simulink model "MotionController_mod"  (Simulink 7.6)
settings: Solver=FixedStepDiscrete  SolverMode=SingleTasking  StartTime=0.0  StopTime=inf  FixedStep=0.02  RelTol=1e-3  SampleTimeConstraint=Specified
undefined symbols (not defined in the file): Compass_Yaw_Kd, Compass_Yaw_Ki, Compass_Yaw_Kp, Depth_Kd, Depth_Ki, Depth_Kp, DiscIntNeverNeededParam, IMU_YawRate_Kd, IMU_YawRate_Ki, IMU_YawRate_Kp, IMU_YVel_Kd, IMU_YVel_Ki, IMU_YVel_Kp, Target_Down_X_Kd, Target_Down_X_Ki, Target_Down_X_Kp, Target_Down_Y_Kd, Target_Down_Y_Ki, Target_Down_Y_Kp, Target_Down_Yaw_Kd, Target_Down_Yaw_Ki, Target_Down_Yaw_Kp, Target_Forward_Y_Kd, Target_Forward_Y_Ki, Target_Forward_Y_Kp, Target_Forward_Yaw_Kd, Target_Forward_Yaw_Ki, Target_Forward_Yaw_Kp, Target_Forward_Z_Kd, Target_Forward_Z_Ki, Target_Forward_Z_Kp, Thruster_Friction_Zero, Thruster_LeftAngled_Gain, Thruster_LeftFwd_Gain, Thruster_RightAngled_Gain, Thruster_RightFwd_Gain, ZVelocity_Neg_Max
libraries: simulink x13, libAUVT x6, neural x1
settings Model: Creator=auvt  LastModifiedBy=auvt  ParamWorkspaceSource=ReferencedWorkspace  TunableVars=Compass_Yaw_Kd,Compass_Yaw_Ki,Compass_Yaw_Kp,Depth_Kd,Depth_Ki,Depth_Kp,Heading_Kd,Heading_Ki,Heading_Kp,IMU_YVel_Kd,IMU_YVel_Ki,IMU_YVel_Kp,IMU_YawRate_Kd,IMU_YawRate_Ki,IMU_YawRate_Kp,Target_Down_X_Kd,Target_Down_X_Ki,Target_Down_X_Kp,Target_Down_Y_Kd,Target_Down_Y_Ki,Target_Down_Y_Kp,Target_Down_Yaw_Kd,Target_Down_Yaw_Ki,Target_Down_Yaw_Kp,Target_Forward_Y_Kd,Target_Forward_Y_Ki,Target_Forward_Y_Kp,Target_Forward_Yaw_Kd,Target_Forward_Yaw_Ki,Target_Forward_Yaw_Kp,Target_Forward_Z_Kd,Target_Forward_Z_Ki,Target_Forward_Z_Kp,Thruster_Friction_Zero,Thruster_LeftAngled_Gain,Thruster_LeftFwd_Gain,Thruster_RightAngled_Gain,Thruster_RightFwd_Gain,ZVelocity_Neg_Max  TunableVarsStorageClass=Auto,Auto,Auto,Auto,Auto,Auto,Auto,Auto,Auto,Auto,Auto,Auto,Auto,Auto,Auto,Auto,Auto,Auto,Auto,Auto,Auto,Auto,Auto,Auto,Auto,Auto,Auto,Auto,Auto,Auto,Auto,Auto,Auto,Auto,Auto,Auto,Auto,Auto,Auto  TunableVarsTypeQualifier=,,,,,,,,,,,,,,,,,,,,,,,,,,,,,,,,,,,,,,
settings MATStruct: SampleTime=0.02  Offset=0  Priority=[1.0]
settings OptimizationCC: InlineParams=on  OptimizeModelRefInitCode=on  LifeSpan=1
settings RTWCC: SystemTargetFile=ert.tlc  GenCodeOnly=on  TemplateMakefile=ert_default_tmf  PostCodeGenCommand=packNGo(buildInfo);  Description=Real-Time Workshop Embedded Coder  GenerateReport=on  ProcessScript=ert_make_rtw_hook  IncludeHyperlinkInReport=on  LaunchReport=on  TargetLang=C++
settings CodeAppCC: IgnoreCustomStorageClasses=off
settings ERTTargetCC: MultiwordLength=2048  GenerateSampleERTMain=on  IncludeMdlTerminateFcn=off  InlinedParameterPlacement=NonHierarchical  ERTCustomFileTemplate=example_file_process.tlc  ConvertIfToSwitch=off

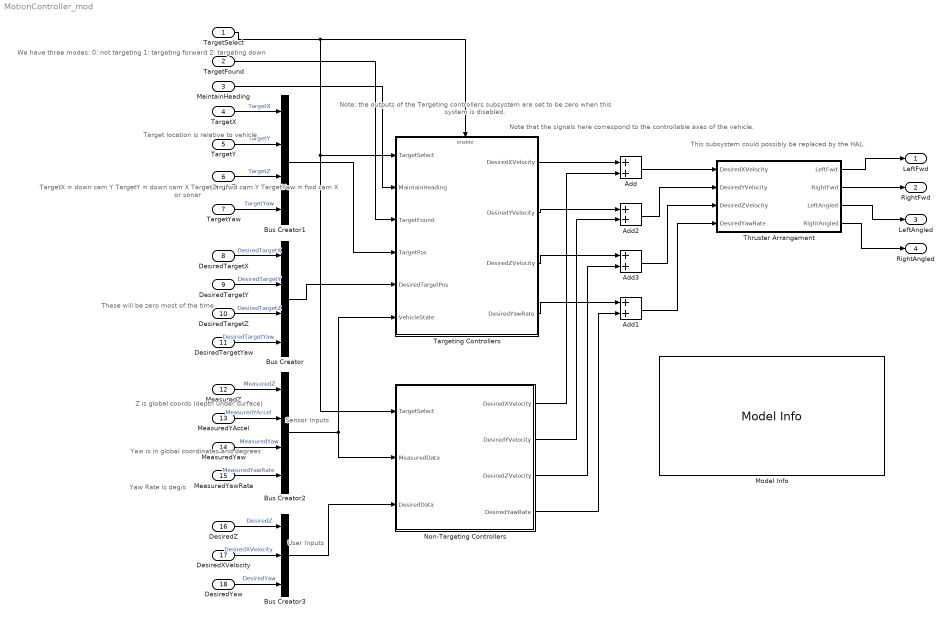
== system MotionController_mod ==
  note: We have three modes:
      |  0: not targeting
      | 1: targeting forward
      | 2: targeting down
  note: Target location
      | is relative to
      | vehicle
  note: Yaw is in global
      | coordinates
      | and degrees
  note: Yaw Rate is deg/s
  note: These will be zero
      | most of the time
  note: Z is global coords
      | (depth under surface)
  note: TargetX = down cam Y
      | TargetY = down cam X
      | TargetZ = fwd cam Y
      | TargetYaw = fwd cam X
      | or sonar
  note: This subsystem could possibly
      |  be replaced by the HAL.
  note: Note that the signals here correspond
      | to the controllable axes of the vehicle.
  note: Sensor
      | Inputs
  note: User
      | Inputs
  note: Note: the outputs of the Targeting controllers
      | subsystem are set to be zero when this
      | system is disabled.
  TargetSelect : Inport  SampleTime=0.02
  TargetFound : Inport  Port=2  SampleTime=0.02
  MaintainHeading : Inport  Port=3
  TargetX : Inport  Port=4
  TargetY : Inport  Port=5
  TargetZ : Inport  Port=6
  TargetYaw : Inport  Port=7
  DesiredTargetX : Inport  Port=8
  DesiredTargetY : Inport  Port=9
  DesiredTargetZ : Inport  Port=10
  DesiredTargetYaw : Inport  Port=11
  MeasuredZ : Inport  Port=12  SampleTime=0.02
  MeasuredYAccel : Inport  Port=13  SampleTime=0.02
  MeasuredYaw : Inport  Port=14  SampleTime=0.02
  MeasuredYawRate : Inport  Port=15
  DesiredZ : Inport  Port=16
  DesiredXVelocity : Inport  Port=17
  DesiredYaw : Inport  Port=18
  Add{,1..3} (4 alike) : Sum
  Bus Creator : BusCreator
  Bus Creator1 : BusCreator
  Bus Creator2 : BusCreator
  Bus Creator3 : BusCreator  Inputs=3
  Model Info : simulink/Model-Wide Utilities/Model Info  SystemSampleTime=-1  InitialBlockCM=None  BlockCM=None  Frame=on  DisplayStringWithTags=|  HorizontalTextAlignment=Left  LeftAlignmentValue=0.02  SourceBlockDiagram=MotionController_mod  TagMaxNumber=20
      | This Model directly controls the
      |  thrusters by using several controllers. 
      |  The controllers are based on current
      |  state information (heading, depth, etc.)
      |  as well as desired state info.
      | 
      | %<LastModifiedBy>
      | %<LastModificationDate>
  Non-Targeting Controllers : Subsystem
  Targeting Controllers : Subsystem  TreatAsAtomicUnit=on
  Thruster Arrangement : Subsystem
  LeftFwd : Outport
  RightFwd : Outport  Port=2
  LeftAngled : Outport  Port=3
  RightAngled : Outport  Port=4
  wires:
  Thruster Arrangement/1(LeftFwd) -> LeftFwd/1
  Thruster Arrangement/2(RightFwd) -> RightFwd/1
  Thruster Arrangement/3(LeftAngled) -> LeftAngled/1
  Thruster Arrangement/4(RightAngled) -> RightAngled/1
  TargetSelect/1 -> Targeting Controllers/Enable, Non-Targeting Controllers/1(TargetSelect), Targeting Controllers/1(TargetSelect)
  TargetFound/1 -> Targeting Controllers/3(TargetFound)
  Add/1 -> Thruster Arrangement/1(DesiredXVelocity)
  Add1/1 -> Thruster Arrangement/4(DesiredYawRate)
  Add2/1 -> Thruster Arrangement/2(DesiredYVelocity)
  Add3/1 -> Thruster Arrangement/3(DesiredZVelocity)
  Targeting Controllers/1(DesiredXVelocity) -> Add/1
  Targeting Controllers/4(DesiredYawRate) -> Add1/1
  Targeting Controllers/2(DesiredYVelocity) -> Add2/1
  Targeting Controllers/3(DesiredZVelocity) -> Add3/1
  Non-Targeting Controllers/2(DesiredYVelocity) -> Add2/2
  Non-Targeting Controllers/4(DesiredYawRate) -> Add1/2
  Non-Targeting Controllers/3(DesiredZVelocity) -> Add3/2
  DesiredTargetX/1 -> Bus Creator/1  "DesiredTargetX"
  DesiredTargetY/1 -> Bus Creator/2  "DesiredTargetY"
  DesiredTargetZ/1 -> Bus Creator/3  "DesiredTargetZ"
  DesiredTargetYaw/1 -> Bus Creator/4  "DesiredTargetYaw"
  TargetX/1 -> Bus Creator1/1  "TargetX"
  TargetY/1 -> Bus Creator1/2  "TargetY"
  TargetZ/1 -> Bus Creator1/3  "TargetZ"
  TargetYaw/1 -> Bus Creator1/4  "TargetYaw"
  Bus Creator1/1 -> Targeting Controllers/4(TargetPos)
  Bus Creator/1 -> Targeting Controllers/5(DesiredTargetPos)
  Non-Targeting Controllers/1(DesiredXVelocity) -> Add/2
  Bus Creator3/1 -> Non-Targeting Controllers/3(DesiredData)
  MeasuredZ/1 -> Bus Creator2/1  "MeasuredZ"
  MeasuredYAccel/1 -> Bus Creator2/2  "MeasuredYAccel"
  MeasuredYaw/1 -> Bus Creator2/3  "MeasuredYaw"
  MeasuredYawRate/1 -> Bus Creator2/4  "MeasuredYawRate"
  DesiredZ/1 -> Bus Creator3/1  "DesiredZ"
  DesiredXVelocity/1 -> Bus Creator3/2  "DesiredXVelocity"
  DesiredYaw/1 -> Bus Creator3/3  "DesiredYaw"
  Bus Creator2/1 -> Targeting Controllers/6(VehicleState), Non-Targeting Controllers/2(MeasuredData)
  MaintainHeading/1 -> Targeting Controllers/2(MaintainHeading)

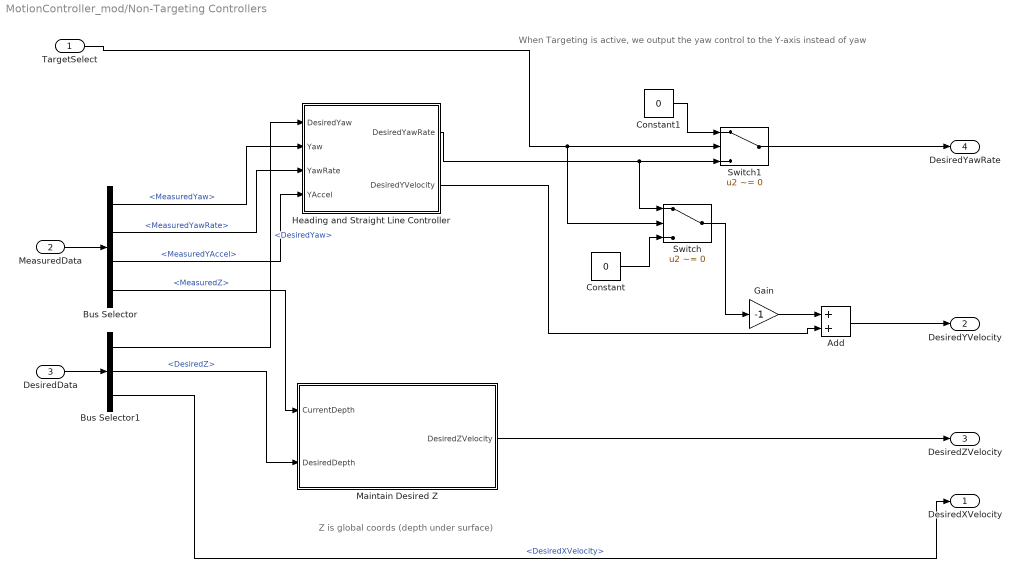
== system MotionController_mod/Non-Targeting Controllers ==
  note: Z is global coords
      | (depth under surface)
  note: When Targeting is active, we output the
      | yaw control to the Y-axis instead of yaw
  TargetSelect : Inport
  MeasuredData : Inport  Port=2
  DesiredData : Inport  Port=3
  Add : Sum
  Bus Selector : BusSelector  OutputSignals=MeasuredYaw,MeasuredYawRate,MeasuredYAccel,MeasuredZ
  Bus Selector1 : BusSelector  OutputSignals=DesiredYaw,DesiredZ,DesiredXVelocity
  Constant : Constant  Value=0
  Constant1 : Constant  Value=0
  Gain : Gain  Gain=-1
  Heading and Straight Line Controller : Subsystem
  "Maintain Desired Z " : Subsystem
      settings: UndoDeleteFcn=Stateflow.SLINSF.SimulinkMan.restorePreDeleteFcn  PreDeleteFcn=Stateflow.SLINSF.SimulinkMan.removePreDeleteFcn
  Switch : Switch  Criteria=u2 ~= 0
  Switch1 : Switch  Criteria=u2 ~= 0
  DesiredXVelocity : Outport
  DesiredYVelocity : Outport  Port=2
  DesiredZVelocity : Outport  Port=3  OutDataTypeStr=double
  DesiredYawRate : Outport  Port=4
  wires:
  Heading and Straight Line Controller/1(DesiredYawRate) -> Switch/1, Switch1/3
  MeasuredData/1 -> Bus Selector/1
  Constant/1 -> Switch/3
  Heading and Straight Line Controller/2(DesiredYVelocity) -> Add/2
  DesiredData/1 -> Bus Selector1/1
  Switch/1 -> Gain/1
  Constant1/1 -> Switch1/1
  Gain/1 -> Add/1
  TargetSelect/1 -> Switch1/2, Switch/2
  Bus Selector/1 -> Heading and Straight Line Controller/2(Yaw)  "<MeasuredYaw>"
  Bus Selector/2 -> Heading and Straight Line Controller/3(YawRate)  "<MeasuredYawRate>"
  Bus Selector/3 -> Heading and Straight Line Controller/4(YAccel)  "<MeasuredYAccel>"
  Bus Selector/4 -> "Maintain Desired Z "/1(CurrentDepth)  "<MeasuredZ>"
  Bus Selector1/1 -> Heading and Straight Line Controller/1(DesiredYaw)  "<DesiredYaw>"
  Bus Selector1/2 -> "Maintain Desired Z "/2(DesiredDepth)  "<DesiredZ>"
  "Maintain Desired Z "/1(DesiredZVelocity) -> DesiredZVelocity/1
  Add/1 -> DesiredYVelocity/1
  Switch1/1 -> DesiredYawRate/1
  Bus Selector1/3 -> DesiredXVelocity/1  "<DesiredXVelocity>"

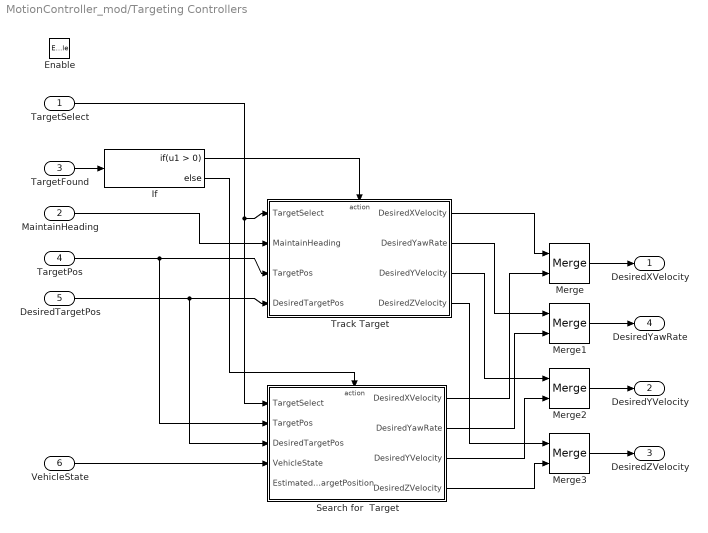
== system MotionController_mod/Targeting Controllers ==
  TargetSelect : Inport
  MaintainHeading : Inport  Port=2
  TargetFound : Inport  Port=3
  TargetPos : Inport  Port=4
  DesiredTargetPos : Inport  Port=5
  VehicleState : Inport  Port=6
  Enable : EnablePort  StatesWhenEnabling=reset
  If : If
  Merge{,1..3} (4 alike) : Merge
  Search for  Target : Subsystem  TreatAsAtomicUnit=on
  Track Target : Subsystem  TreatAsAtomicUnit=on
  DesiredXVelocity : Outport  OutputWhenDisabled=reset  InitialOutput=0
  DesiredYVelocity : Outport  Port=2  OutputWhenDisabled=reset  InitialOutput=0
  DesiredZVelocity : Outport  Port=3  OutDataTypeStr=double  OutputWhenDisabled=reset  InitialOutput=0
  DesiredYawRate : Outport  Port=4  OutputWhenDisabled=reset  InitialOutput=0
  wires:
  TargetFound/1 -> If/1
  If/1 -> Track Target/Action
  TargetPos/1 -> Track Target/3(TargetPos), Search for  Target/2(TargetPos)
  DesiredTargetPos/1 -> Track Target/4(DesiredTargetPos), Search for  Target/3(DesiredTargetPos)
  If/2 -> Search for  Target/Action
  VehicleState/1 -> Search for  Target/4(VehicleState)
  Track Target/1(DesiredXVelocity) -> Merge/1
  Track Target/2(DesiredYawRate) -> Merge1/1
  Track Target/3(DesiredYVelocity) -> Merge2/1
  Track Target/4(DesiredZVelocity) -> Merge3/1
  Search for  Target/1(DesiredXVelocity) -> Merge/2
  Search for  Target/2(DesiredYawRate) -> Merge1/2
  Search for  Target/3(DesiredYVelocity) -> Merge2/2
  Search for  Target/4(DesiredZVelocity) -> Merge3/2
  Merge/1 -> DesiredXVelocity/1
  Merge1/1 -> DesiredYawRate/1
  Merge2/1 -> DesiredYVelocity/1
  Merge3/1 -> DesiredZVelocity/1
  TargetSelect/1 -> Track Target/1(TargetSelect), Search for  Target/1(TargetSelect)
  MaintainHeading/1 -> Track Target/2(MaintainHeading)

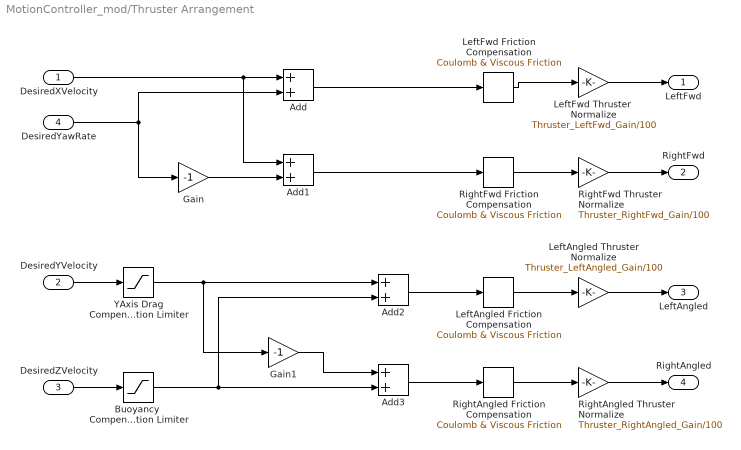
== system MotionController_mod/Thruster Arrangement ==
  DesiredXVelocity : Inport
  DesiredYVelocity : Inport  Port=2
  DesiredZVelocity : Inport  Port=3
  DesiredYawRate : Inport  Port=4
  Add{,1..3} (4 alike) : Sum
  Buoyancy  Compensation Limiter : Saturate  UpperLimit=100  LowerLimit=ZVelocity_Neg_Max
  Gain : Gain  Gain=-1
  Gain1 : Gain  Gain=-1
  LeftAngled Friction Compensation : simulink/Discontinuities/Coulomb & Viscous Friction  SystemSampleTime=-1  offset=Thruster_Friction_Zero  gain=(100-Thruster_Friction_Zero)/100
  LeftAngled Thruster Normalize : Gain  Gain=Thruster_LeftAngled_Gain/100
  LeftFwd Friction Compensation : simulink/Discontinuities/Coulomb & Viscous Friction  SystemSampleTime=-1  offset=Thruster_Friction_Zero  gain=(100-Thruster_Friction_Zero)/100
  LeftFwd Thruster  Normalize : Gain  Gain=Thruster_LeftFwd_Gain/100
  RightAngled Friction Compensation : simulink/Discontinuities/Coulomb & Viscous Friction  SystemSampleTime=-1  offset=Thruster_Friction_Zero  gain=(100-Thruster_Friction_Zero)/100
  RightAngled Thruster Normalize : Gain  Gain=Thruster_RightAngled_Gain/100
  RightFwd Friction Compensation : simulink/Discontinuities/Coulomb & Viscous Friction  SystemSampleTime=-1  offset=Thruster_Friction_Zero  gain=(100-Thruster_Friction_Zero)/100
  RightFwd Thruster Normalize : Gain  Gain=Thruster_RightFwd_Gain/100
  YAxis Drag Compensation Limiter : Saturate  UpperLimit=100  LowerLimit=-100  LinearizeAsGain=off
  LeftFwd : Outport
  RightFwd : Outport  Port=2
  LeftAngled : Outport  Port=3
  RightAngled : Outport  Port=4
  wires:
  DesiredYawRate/1 -> Gain/1, Add/2
  LeftFwd Thruster  Normalize/1 -> LeftFwd/1
  RightFwd Thruster Normalize/1 -> RightFwd/1
  LeftFwd Friction Compensation/1 -> LeftFwd Thruster  Normalize/1
  RightFwd Friction Compensation/1 -> RightFwd Thruster Normalize/1
  LeftAngled Thruster Normalize/1 -> LeftAngled/1
  RightAngled Thruster Normalize/1 -> RightAngled/1
  DesiredXVelocity/1 -> Add1/1, Add/1
  Add/1 -> LeftFwd Friction Compensation/1
  Add1/1 -> RightFwd Friction Compensation/1
  DesiredYVelocity/1 -> YAxis Drag Compensation Limiter/1
  LeftAngled Friction Compensation/1 -> LeftAngled Thruster Normalize/1
  DesiredZVelocity/1 -> Buoyancy  Compensation Limiter/1
  RightAngled Friction Compensation/1 -> RightAngled Thruster Normalize/1
  Add2/1 -> LeftAngled Friction Compensation/1
  Add3/1 -> RightAngled Friction Compensation/1
  YAxis Drag Compensation Limiter/1 -> Add2/1, Gain1/1
  Gain1/1 -> Add3/1
  Buoyancy  Compensation Limiter/1 -> Add2/2, Add3/2
  Gain/1 -> Add1/2

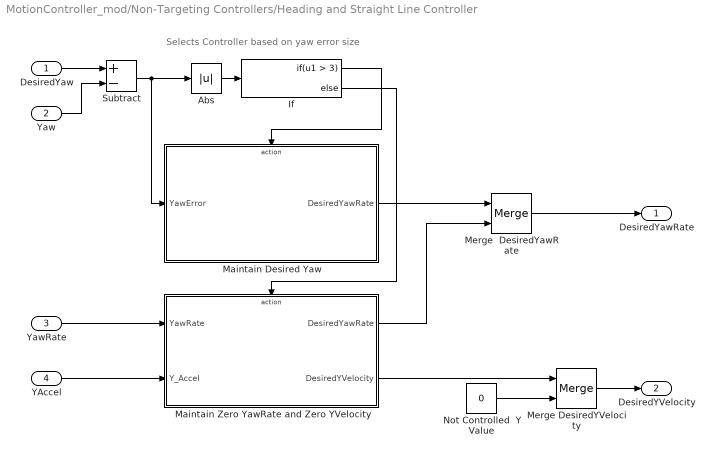
== system MotionController_mod/Non-Targeting Controllers/Heading and Straight Line Controller ==
  note: Selects Controller based on yaw error size
  DesiredYaw : Inport
  Yaw : Inport  Port=2
  YawRate : Inport  Port=3
  YAccel : Inport  Port=4
  Abs : Abs
  If : If  IfExpression=u1 > 3
  Maintain Desired Yaw : Subsystem  TreatAsAtomicUnit=on
  Maintain Zero YawRate and Zero YVelocity : Subsystem
      settings: UndoDeleteFcn=Stateflow.SLINSF.SimulinkMan.restorePreDeleteFcn  PreDeleteFcn=Stateflow.SLINSF.SimulinkMan.removePreDeleteFcn
  Merge DesiredYVelocity : Merge
  Merge  DesiredYawRate : Merge
  Not Controlled  Y Value : Constant  Value=0
  Subtract : Sum  Inputs=+-
  DesiredYawRate : Outport
  DesiredYVelocity : Outport  Port=2
  wires:
  If/1 -> Maintain Desired Yaw/Action
  Subtract/1 -> Abs/1, Maintain Desired Yaw/1(YawError)
  Abs/1 -> If/1
  Maintain Zero YawRate and Zero YVelocity/1(DesiredYawRate) -> Merge  DesiredYawRate/2
  Not Controlled  Y Value/1 -> Merge DesiredYVelocity/2
  Maintain Zero YawRate and Zero YVelocity/2(DesiredYVelocity) -> Merge DesiredYVelocity/1
  Maintain Desired Yaw/1(DesiredYawRate) -> Merge  DesiredYawRate/1
  If/2 -> Maintain Zero YawRate and Zero YVelocity/Action
  DesiredYaw/1 -> Subtract/1
  Yaw/1 -> Subtract/2
  Merge  DesiredYawRate/1 -> DesiredYawRate/1
  YawRate/1 -> Maintain Zero YawRate and Zero YVelocity/1(YawRate)
  YAccel/1 -> Maintain Zero YawRate and Zero YVelocity/2(Y_Accel)
  Merge DesiredYVelocity/1 -> DesiredYVelocity/1

== system MotionController_mod/Non-Targeting Controllers/Maintain Desired Z  ==
  note: Error
  CurrentDepth : Inport  OutDataTypeStr=double
  DesiredDepth : Inport  Port=2  OutDataTypeStr=double
  Add : Sum  Inputs=+-  OutDataTypeStr=double
  PID Controller Depth S3 : Subsystem  Description=PID
  DesiredZVelocity : Outport  OutDataTypeStr=double
  wires:
  Add/1 -> PID Controller Depth S3/1(e)
  PID Controller Depth S3/1(u) -> DesiredZVelocity/1
  CurrentDepth/1 -> Add/2
  DesiredDepth/1 -> Add/1

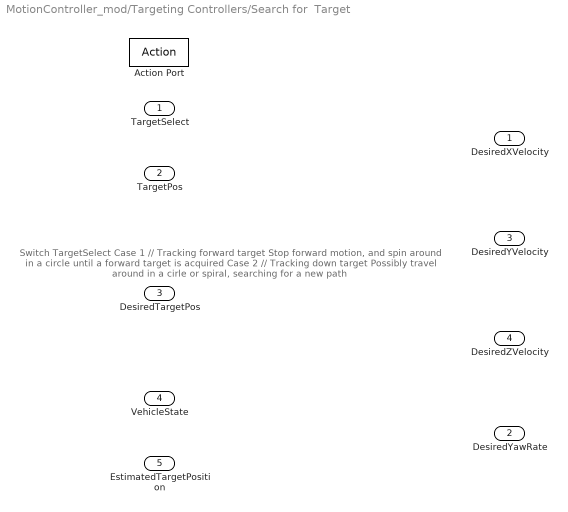
== system MotionController_mod/Targeting Controllers/Search for  Target ==
  note: Switch TargetSelect
      |   Case 1 // Tracking forward target
      |     Stop forward motion, and spin around in a circle
      |     until a forward target is acquired
      |   Case 2 // Tracking down target
      |     Possibly travel around in a cirle or spiral,
      |     searching for a new path
  TargetSelect : Inport
  TargetPos : Inport  Port=2
  DesiredTargetPos : Inport  Port=3
  VehicleState : Inport  Port=4
  EstimatedTargetPosition : Inport  Port=5
  Action Port : ActionPort  ActionType=else
  DesiredXVelocity : Outport
  DesiredYawRate : Outport  Port=2
  DesiredYVelocity : Outport  Port=3
  DesiredZVelocity : Outport  Port=4  OutDataTypeStr=double

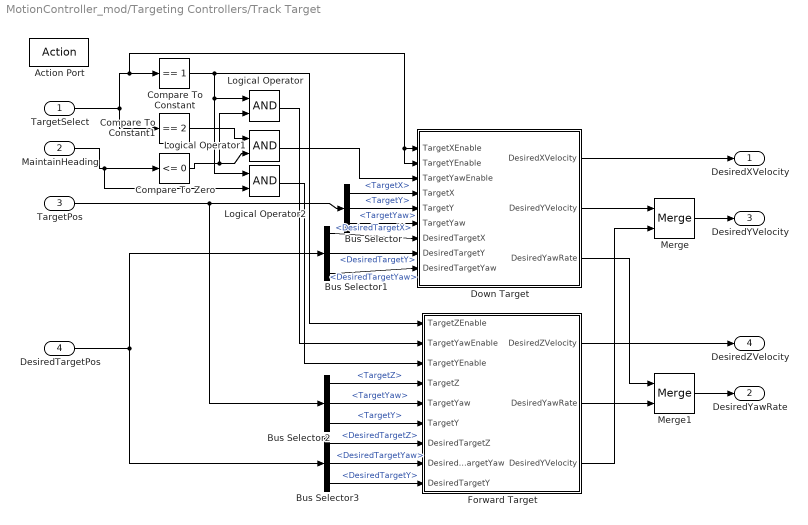
== system MotionController_mod/Targeting Controllers/Track Target ==
  TargetSelect : Inport
  MaintainHeading : Inport  Port=2
  TargetPos : Inport  Port=3
  DesiredTargetPos : Inport  Port=4
  Action Port : ActionPort  ActionType=then
  Bus Selector : BusSelector  OutputSignals=TargetX,TargetY,TargetYaw
  Bus Selector1 : BusSelector  OutputSignals=DesiredTargetX,DesiredTargetY,DesiredTargetYaw
  Bus Selector2 : BusSelector  OutputSignals=TargetZ,TargetYaw,TargetY
  Bus Selector3 : BusSelector  OutputSignals=DesiredTargetZ,DesiredTargetYaw,DesiredTargetY
  Compare To Constant : simulink/Logic and Bit Operations/Compare To Constant  SystemSampleTime=-1  relop===  const=1  LogicOutDataTypeMode=uint8
  Compare To Constant1 : simulink/Logic and Bit Operations/Compare To Constant  SystemSampleTime=-1  relop===  const=2  LogicOutDataTypeMode=uint8
  Compare To Zero : simulink/Logic and Bit Operations/Compare To Zero  SystemSampleTime=-1  relop=<=  LogicOutDataTypeMode=uint8
  Down Target : Subsystem
  Forward Target : Subsystem
  Logical Operator : Logic  AllPortsSameDT=off  OutDataTypeStr=boolean
  Logical Operator1 : Logic  AllPortsSameDT=off  OutDataTypeStr=boolean
  Logical Operator2 : Logic  AllPortsSameDT=off  OutDataTypeStr=boolean
  Merge : Merge
  Merge1 : Merge
  DesiredXVelocity : Outport
  DesiredYawRate : Outport  Port=2
  DesiredYVelocity : Outport  Port=3
  DesiredZVelocity : Outport  Port=4  OutDataTypeStr=double
  wires:
  TargetPos/1 -> Bus Selector/1, Bus Selector2/1
  DesiredTargetPos/1 -> Bus Selector1/1, Bus Selector3/1
  Forward Target/1(DesiredZVelocity) -> DesiredZVelocity/1
  Down Target/1(DesiredXVelocity) -> DesiredXVelocity/1
  Down Target/2(DesiredYVelocity) -> Merge/1
  Down Target/3(DesiredYawRate) -> Merge1/1
  Forward Target/2(DesiredYawRate) -> Merge1/2
  Forward Target/3(DesiredYVelocity) -> Merge/2
  Merge/1 -> DesiredYVelocity/1
  Merge1/1 -> DesiredYawRate/1
  Bus Selector/1 -> Down Target/4(TargetX)  "<TargetX>"
  Bus Selector/2 -> Down Target/5(TargetY)  "<TargetY>"
  Bus Selector/3 -> Down Target/6(TargetYaw)  "<TargetYaw>"
  Bus Selector1/1 -> Down Target/7(DesiredTargetX)  "<DesiredTargetX>"
  Bus Selector1/2 -> Down Target/8(DesiredTargetY)  "<DesiredTargetY>"
  Bus Selector1/3 -> Down Target/9(DesiredTargetYaw)  "<DesiredTargetYaw>"
  Bus Selector2/1 -> Forward Target/4(TargetZ)  "<TargetZ>"
  Bus Selector2/2 -> Forward Target/5(TargetYaw)  "<TargetYaw>"
  Bus Selector2/3 -> Forward Target/6(TargetY)  "<TargetY>"
  Bus Selector3/1 -> Forward Target/7(DesiredTargetZ)  "<DesiredTargetZ>"
  Bus Selector3/2 -> Forward Target/8(DesiredTargetYaw)  "<DesiredTargetYaw>"
  Bus Selector3/3 -> Forward Target/9(DesiredTargetY)  "<DesiredTargetY>"
  MaintainHeading/1 -> Compare To Zero/1, Logical Operator2/2
  TargetSelect/1 -> Compare To Constant1/1, Compare To Constant/1, Down Target/2(TargetYEnable), Down Target/1(TargetXEnable)
  Compare To Zero/1 -> Logical Operator/2, Logical Operator1/2
  Compare To Constant1/1 -> Logical Operator1/1
  Compare To Constant/1 -> Logical Operator/1, Logical Operator2/1, Forward Target/1(TargetZEnable)
  Logical Operator2/1 -> Forward Target/3(TargetYEnable)
  Logical Operator/1 -> Forward Target/2(TargetYawEnable)
  Logical Operator1/1 -> Down Target/3(TargetYawEnable)

== system MotionController_mod/Non-Targeting Controllers/Heading and Straight Line Controller/Maintain Desired Yaw ==
  note: Error Shaping corrects for controller
      | behavior over large error values vs.
      | small errors.
  note: Error Ranging puts the error in
      | the range -180 to +180
  note: Yaw = Heading
  note: Error = Desired - Measured
  YawError : Inport  PortDimensions=1
  Action Port : ActionPort  InitializeStates=reset  ActionType=then
  Error Shaping : Subsystem
  Error Shifting and Range Checking : Subsystem
  PID Controller Heading : Subsystem  Description=PID
  DesiredYawRate : Outport
  wires:
  YawError/1 -> Error Shifting and Range Checking/1(Raw Error)  "YawError"
  Error Shifting and Range Checking/1(Ranged Error) -> Error Shaping/1(Ranged Error)
  Error Shaping/1(Shaped Error) -> PID Controller Heading/1(e)
  PID Controller Heading/1(u) -> DesiredYawRate/1

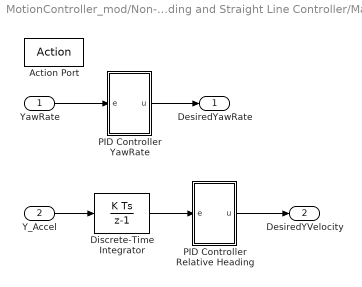
== system MotionController_mod/Non-Targeting Controllers/Heading and Straight Line Controller/Maintain Zero YawRate and Zero YVelocity ==
  YawRate : Inport
  Y_Accel : Inport  Port=2
  Action Port : ActionPort  InitializeStates=reset  ActionType=else
  Discrete-Time Integrator : DiscreteIntegrator  SampleTime=-1  LimitOutput=on  UpperSaturationLimit=10  LowerSaturationLimit=-10  IgnoreLimit=on  ICPrevOutput=DiscIntNeverNeededParam  ICPrevScaledInput=DiscIntNeverNeededParam
  PID Controller Relative Heading : Subsystem  Description=PID
  PID Controller YawRate : Subsystem  Description=PID
  DesiredYawRate : Outport
  DesiredYVelocity : Outport  Port=2
  wires:
  Y_Accel/1 -> Discrete-Time Integrator/1
  YawRate/1 -> PID Controller YawRate/1(e)
  PID Controller Relative Heading/1(u) -> DesiredYVelocity/1
  PID Controller YawRate/1(u) -> DesiredYawRate/1
  Discrete-Time Integrator/1 -> PID Controller Relative Heading/1(e)

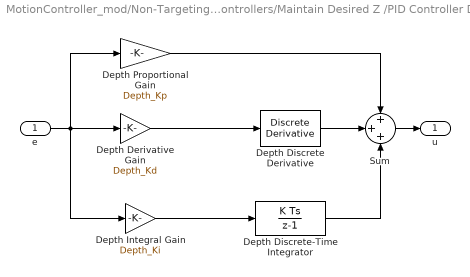
== system MotionController_mod/Non-Targeting Controllers/Maintain Desired Z /PID Controller Depth S3 ==
  e : Inport
  Depth Derivative Gain : Gain  Gain=Depth_Kd
  Depth Discrete Derivative : simulink/Discrete/Discrete Derivative  SystemSampleTime=-1  gainval=1  ICPrevScaledInput=0.0  OutMin=[]  OutMax=[]  OutDataType=fixdt(1, 16)  OutScaling=2^-10  DoSatur=on
  Depth Discrete-Time Integrator : DiscreteIntegrator  gainval=1  SampleTime=-1  LimitOutput=on  UpperSaturationLimit=10  LowerSaturationLimit=-10  ICPrevOutput=DiscIntNeverNeededParam  ICPrevScaledInput=DiscIntNeverNeededParam
  Depth Integral Gain : Gain  Gain=Depth_Ki
  Depth Proportional Gain : Gain  Gain=Depth_Kp
  Sum : Sum  Inputs=+++  SaturateOnIntegerOverflow=on  InputSameDT=on  OutDataTypeStr=Inherit: Same as first input
  u : Outport
  wires:
  e/1 -> Depth Proportional Gain/1, Depth Derivative Gain/1, Depth Integral Gain/1
  Depth Discrete-Time Integrator/1 -> Sum/3
  Depth Proportional Gain/1 -> Sum/1
  Sum/1 -> u/1
  Depth Discrete Derivative/1 -> Sum/2
  Depth Derivative Gain/1 -> Depth Discrete Derivative/1
  Depth Integral Gain/1 -> Depth Discrete-Time Integrator/1

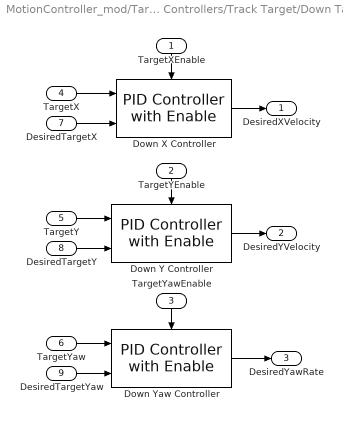
== system MotionController_mod/Targeting Controllers/Track Target/Down Target ==
  TargetXEnable : Inport
  TargetYEnable : Inport  Port=2
  TargetYawEnable : Inport  Port=3
  TargetX : Inport  Port=4
  TargetY : Inport  Port=5
  TargetYaw : Inport  Port=6
  DesiredTargetX : Inport  Port=7
  DesiredTargetY : Inport  Port=8
  DesiredTargetYaw : Inport  Port=9
  Down X Controller : libAUVT/PID Controller with Enable  SystemSampleTime=-1  Kp=Target_Down_X_Kp  Ki=Target_Down_X_Ki  Kd=Target_Down_X_Kd
  Down Y Controller : libAUVT/PID Controller with Enable  SystemSampleTime=-1  Kp=Target_Down_Y_Kp  Ki=Target_Down_Y_Ki  Kd=Target_Down_Y_Kd
  Down Yaw Controller : libAUVT/PID Controller with Enable  SystemSampleTime=-1  Kp=Target_Down_Yaw_Kp  Ki=Target_Down_Yaw_Ki  Kd=Target_Down_Yaw_Kd
  DesiredXVelocity : Outport  OutputWhenDisabled=reset  InitialOutput=0
  DesiredYVelocity : Outport  Port=2  OutputWhenDisabled=reset  InitialOutput=0
  DesiredYawRate : Outport  Port=3  OutputWhenDisabled=reset  InitialOutput=0
  wires:
  TargetYaw/1 -> Down Yaw Controller/1
  DesiredTargetYaw/1 -> Down Yaw Controller/2
  TargetY/1 -> Down Y Controller/1
  DesiredTargetY/1 -> Down Y Controller/2
  TargetX/1 -> Down X Controller/1
  DesiredTargetX/1 -> Down X Controller/2
  TargetXEnable/1 -> Down X Controller/Enable
  TargetYEnable/1 -> Down Y Controller/Enable
  TargetYawEnable/1 -> Down Yaw Controller/Enable
  Down X Controller/1 -> DesiredXVelocity/1
  Down Y Controller/1 -> DesiredYVelocity/1
  Down Yaw Controller/1 -> DesiredYawRate/1

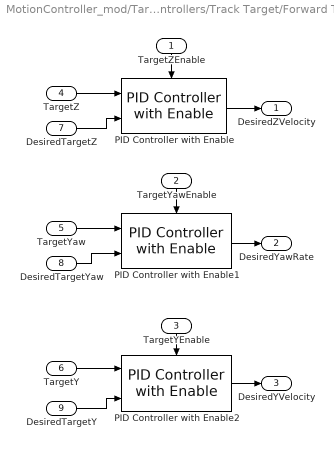
== system MotionController_mod/Targeting Controllers/Track Target/Forward Target ==
  TargetZEnable : Inport
  TargetYawEnable : Inport  Port=2
  TargetYEnable : Inport  Port=3
  TargetZ : Inport  Port=4
  TargetYaw : Inport  Port=5
  TargetY : Inport  Port=6
  DesiredTargetZ : Inport  Port=7
  DesiredTargetYaw : Inport  Port=8
  DesiredTargetY : Inport  Port=9
  PID Controller with Enable : libAUVT/PID Controller with Enable  SystemSampleTime=-1  Kp=Target_Forward_Z_Kp  Ki=Target_Forward_Z_Ki  Kd=Target_Forward_Z_Kd
  PID Controller with Enable1 : libAUVT/PID Controller with Enable  SystemSampleTime=-1  Kp=Target_Forward_Yaw_Kp  Ki=Target_Forward_Yaw_Ki  Kd=Target_Forward_Yaw_Kd
  PID Controller with Enable2 : libAUVT/PID Controller with Enable  SystemSampleTime=-1  Kp=Target_Forward_Y_Kp  Ki=Target_Forward_Y_Ki  Kd=Target_Forward_Y_Kd
  DesiredZVelocity : Outport  OutputWhenDisabled=reset  InitialOutput=0
  DesiredYawRate : Outport  Port=2  OutputWhenDisabled=reset  InitialOutput=0
  DesiredYVelocity : Outport  Port=3  OutputWhenDisabled=reset  InitialOutput=0
  wires:
  PID Controller with Enable/1 -> DesiredZVelocity/1
  DesiredTargetZ/1 -> PID Controller with Enable/2
  PID Controller with Enable1/1 -> DesiredYawRate/1
  TargetZEnable/1 -> PID Controller with Enable/Enable
  TargetYawEnable/1 -> PID Controller with Enable1/Enable
  TargetY/1 -> PID Controller with Enable2/1
  PID Controller with Enable2/1 -> DesiredYVelocity/1
  DesiredTargetY/1 -> PID Controller with Enable2/2
  TargetYEnable/1 -> PID Controller with Enable2/Enable
  TargetZ/1 -> PID Controller with Enable/1
  TargetYaw/1 -> PID Controller with Enable1/1
  DesiredTargetYaw/1 -> PID Controller with Enable1/2

== system MotionController_mod/Non-Targeting Controllers/Heading and Straight Line Controller/Maintain Desired Yaw/Error Shaping ==
  note: Error
  Ranged Error : Inport
  1/Saturation Angle : Gain  Gain=1/45
  DocBlock : simulink/Model-Wide Utilities/DocBlock  SystemSampleTime=-1  DocumentType=Text
  Saturation Angle : Gain  Gain=45
  tansig1 : neural/Transfer Functions/tansig  SystemSampleTime=-1
  Shaped Error : Outport
  wires:
  Ranged Error/1 -> 1/Saturation Angle/1
  1/Saturation Angle/1 -> tansig1/1
  tansig1/1 -> Saturation Angle/1
  Saturation Angle/1 -> Shaped Error/1

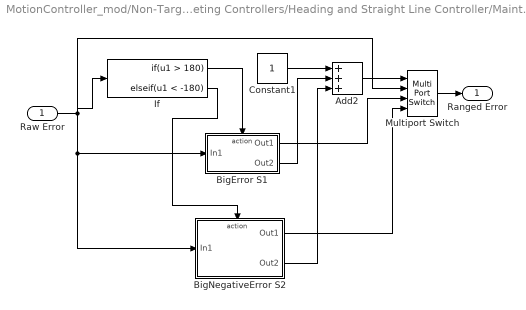
== system MotionController_mod/Non-Targeting Controllers/Heading and Straight Line Controller/Maintain Desired Yaw/Error Shifting and Range Checking ==
  Raw Error : Inport
  Add2 : Sum  Inputs=+++
  BigError S1 : Subsystem  TreatAsAtomicUnit=on
  BigNegativeError S2 : Subsystem  TreatAsAtomicUnit=on
  Constant1 : Constant  SampleTime=-1
  If : If  IfExpression=u1 > 180  ElseIfExpressions=u1 < -180  ShowElse=off
  Multiport Switch : MultiPortSwitch  zeroidx=off
  Ranged Error : Outport
  wires:
  If/1 -> BigError S1/Action
  If/2 -> BigNegativeError S2/Action
  BigError S1/1(Out1) -> Multiport Switch/3
  BigNegativeError S2/1(Out1) -> Multiport Switch/4
  Constant1/1 -> Add2/1
  BigError S1/2(Out2) -> Add2/2
  BigNegativeError S2/2(Out2) -> Add2/3
  Add2/1 -> Multiport Switch/1
  Raw Error/1 -> Multiport Switch/2, BigNegativeError S2/1(In1), BigError S1/1(In1), If/1
  Multiport Switch/1 -> Ranged Error/1

== system MotionController_mod/Non-Targeting Controllers/Heading and Straight Line Controller/Maintain Desired Yaw/PID Controller Heading ==
  e : Inport
  Heading Derivative Gain : Gain  Gain=Compass_Yaw_Kd
  Heading Discrete Derivative : simulink/Discrete/Discrete Derivative  SystemSampleTime=-1  gainval=1  ICPrevScaledInput=0.0  OutMin=[]  OutMax=[]  OutDataType=fixdt(1, 16)  OutScaling=2^-10  DoSatur=off
  Heading Discrete-Time Integrator : DiscreteIntegrator  gainval=1  SampleTime=-1  LimitOutput=on  UpperSaturationLimit=15  LowerSaturationLimit=-15  ICPrevOutput=DiscIntNeverNeededParam  ICPrevScaledInput=DiscIntNeverNeededParam
  Heading Integral Gain : Gain  Gain=Compass_Yaw_Ki
  Heading Proportional Gain : Gain  Gain=Compass_Yaw_Kp
  Sum : Sum  Inputs=+++  SaturateOnIntegerOverflow=on  InputSameDT=on  OutDataTypeStr=Inherit: Same as first input
  u : Outport
  wires:
  e/1 -> Heading Proportional Gain/1, Heading Derivative Gain/1, Heading Integral Gain/1
  Heading Discrete-Time Integrator/1 -> Sum/3
  Heading Proportional Gain/1 -> Sum/1
  Sum/1 -> u/1
  Heading Discrete Derivative/1 -> Sum/2
  Heading Derivative Gain/1 -> Heading Discrete Derivative/1
  Heading Integral Gain/1 -> Heading Discrete-Time Integrator/1

== system MotionController_mod/Non-Targeting Controllers/Heading and Straight Line Controller/Maintain Zero YawRate and Zero YVelocity/PID Controller Relative Heading ==
  e : Inport
  Depth Discrete Derivative : simulink/Discrete/Discrete Derivative  SystemSampleTime=-1  gainval=1  ICPrevScaledInput=0.0  OutMin=[]  OutMax=[]  OutDataType=fixdt(1, 16)  OutScaling=2^-10  DoSatur=on
  Depth Discrete-Time Integrator : DiscreteIntegrator  gainval=1  SampleTime=-1  LimitOutput=on  UpperSaturationLimit=10  LowerSaturationLimit=-10  ICPrevOutput=DiscIntNeverNeededParam  ICPrevScaledInput=DiscIntNeverNeededParam
  Sum : Sum  Inputs=+++  SaturateOnIntegerOverflow=on  InputSameDT=on  OutDataTypeStr=Inherit: Same as first input
  Y-Accelerometer Derivative Gain : Gain  Gain=IMU_YVel_Kd
  Y-Accelerometer Integral Gain : Gain  Gain=IMU_YVel_Ki
  Y-Accelerometer Proportional Gain : Gain  Gain=IMU_YVel_Kp
  u : Outport
  wires:
  e/1 -> Y-Accelerometer Proportional Gain/1, Y-Accelerometer Derivative Gain/1, Y-Accelerometer Integral Gain/1
  Depth Discrete-Time Integrator/1 -> Sum/3
  Y-Accelerometer Proportional Gain/1 -> Sum/1
  Sum/1 -> u/1
  Depth Discrete Derivative/1 -> Sum/2
  Y-Accelerometer Derivative Gain/1 -> Depth Discrete Derivative/1
  Y-Accelerometer Integral Gain/1 -> Depth Discrete-Time Integrator/1

== system MotionController_mod/Non-Targeting Controllers/Heading and Straight Line Controller/Maintain Zero YawRate and Zero YVelocity/PID Controller YawRate ==
  e : Inport
  Heading Discrete Derivative : simulink/Discrete/Discrete Derivative  SystemSampleTime=-1  gainval=1  ICPrevScaledInput=0.0  OutMin=[]  OutMax=[]  OutDataType=fixdt(1, 16)  OutScaling=2^-10  DoSatur=off
  Heading Discrete-Time Integrator : DiscreteIntegrator  gainval=1  SampleTime=-1  LimitOutput=on  UpperSaturationLimit=15  LowerSaturationLimit=-15  ICPrevOutput=DiscIntNeverNeededParam  ICPrevScaledInput=DiscIntNeverNeededParam
  Sum : Sum  Inputs=+++  SaturateOnIntegerOverflow=on  InputSameDT=on  OutDataTypeStr=Inherit: Same as first input
  YawRate Derivative Gain : Gain  Gain=IMU_YawRate_Kd
  YawRate Integral Gain : Gain  Gain=IMU_YawRate_Ki
  YawRate Proportional Gain : Gain  Gain=IMU_YawRate_Kp
  u : Outport
  wires:
  e/1 -> YawRate Proportional Gain/1, YawRate Derivative Gain/1, YawRate Integral Gain/1
  Heading Discrete-Time Integrator/1 -> Sum/3
  YawRate Proportional Gain/1 -> Sum/1
  Sum/1 -> u/1
  Heading Discrete Derivative/1 -> Sum/2
  YawRate Derivative Gain/1 -> Heading Discrete Derivative/1
  YawRate Integral Gain/1 -> Heading Discrete-Time Integrator/1

== system MotionController_mod/Non-Targeting Controllers/Heading and Straight Line Controller/Maintain Desired Yaw/Error Shifting and Range Checking/BigError S1 ==
  In1 : Inport
  Action Port : ActionPort  PropagateVarSize=During execution  ActionType=then
  Add : Sum  Inputs=+-
  Constant : Constant  Value=360  SampleTime=-1
  Constant1 : Constant  SampleTime=-1
  Out1 : Outport
  Out2 : Outport  Port=2  OutputWhenDisabled=reset  InitialOutput=[0]
  wires:
  In1/1 -> Add/1
  Constant/1 -> Add/2
  Add/1 -> Out1/1
  Constant1/1 -> Out2/1

== system MotionController_mod/Non-Targeting Controllers/Heading and Straight Line Controller/Maintain Desired Yaw/Error Shifting and Range Checking/BigNegativeError S2 ==
  In1 : Inport
  Action Port : ActionPort  PropagateVarSize=During execution  ActionType=elseif
  Add : Sum
  Constant : Constant  Value=360  SampleTime=-1
  Constant1 : Constant  Value=2  SampleTime=-1
  Out1 : Outport
  Out2 : Outport  Port=2  OutputWhenDisabled=reset  InitialOutput=[0]
  wires:
  In1/1 -> Add/1
  Constant/1 -> Add/2
  Add/1 -> Out1/1
  Constant1/1 -> Out2/1
